simulink model "radiator model"  (R2023b)
settings: Solver=VariableStepAuto  StartTime=0.0  StopTime=1300  RelTol=1e-3  AbsTol=1e-3  EnableMultiTasking=on
PreLoadFcn:
  | %  Radiator tubes
  | n_tubes      = 20;                % Number of tubes
  | w_radiator  = 0.025;           % Radiator width [m]
  | h_tube        = 0.0015;         % Tube height [m]
  | L_tube        = 0.45;             % Tube length [m]
  | 
  | % Radiator fins
  | delta_fin     = 1e-4;           % Fin thickness [m]
  | w_fin           = 0.002;          % Fin width [m]
  | h_fin           = 0.012;            % Fin height
  | 
  | 
  | % Fluid jacket
  | Re_TLU   = [6, 8, 12, 14, 16]' .* 1e4;  % Reynolds number vector
  | Pr_TLU   = [2, 4, 6, 8, 10];                  % Prandtl number vector
  | 
  | % Air
  | rho_air          = 1.2;       % Density [kg/m^3]
  | cp_air            = 1004;   % Specific heat [J/kg/K]
  | vel_air_nom = 1;         % Nominal velocity [m/s]
  | HC_nom       = 100;     % Nominal heat transfer coefficient [W/(K*m^2)]
  | HC_min        = 10;       % Minimum heat transfer coefficient [W/(K*m^2)]
InitFcn:
  | % Radiator fins
  | n_fin_rows  = n_tubes - 1;   % Number of fin rows
  | n_fins         = n_fin_rows  * (L_tube / w_fin);   % Total number of fins
  | 
  | % Heat transfer surface area
  | area_primary = 2 * L_tube * w_radiator * (n_fin_rows) - 2 * delta_fin * w_radiator * n_fins + 2 * h_fin * w_radiator * n_fin_rows + 2 * h_tube * n_tubes * L_tube;
  | area_fins        = n_fins * (h_fin-delta_fin) * w_radiator * 2;
  | 
  | % Air
  | area_air = n_fins * h_fin * w_fin;      % Cross-sectional area [m^2]
  | 
  | % Fluid jacket
  | Nu_TLU  = 0.3.* Re_TLU .^ 0.8 * Pr_TLU .* 0.33;  %  Nusselt number table
libraries: fl_lib x13, nesl_utility x9, SimscapeFluids_lib x4
(part 1 of 3)
CloseFcn:
  | try,close(h1_EngineCoolingSystem),end
  | clear h1_EngineCoolingSystem
  | 
  | try,close(h2_EngineCoolingSystem),end
  | clear h2_EngineCoolingSystem
  | 
  | try,close(h3_EngineCoolingSystem),end
  | clear h3_EngineCoolingSystem
  | 
  | try,close(h4_EngineCoolingSystem),end
  | clear h4_EngineCoolingSystem
  | 
  | clear Eng_speed Eng_torque Fan_volt Veh_speed
  | clear n_tubes w_radiator h_tube L_tube
  | clear n_fin_rows delta_fin w_fin h_fin n_fins
  | clear area_primary area_fins
  | clear Re_TLU Pr_TLU Nu_TLU
  | clear rho_air cp_air area_air
  | clear vel_air_nom HC_nom HC_min
  | clear simlog_EngineCoolingSystem yout tout
  | clear logsout_EngineCoolingSystem
Description:
  | Engine Cooling System
settings Model: Creator=The MathWorks, Inc.  LastModifiedBy=Pranjal
settings SolverCC: AutoScaleAbsTol=off  MaxConsecutiveMinStep=2  AlgebraicLoopSolver=TrustRegion  MaxZcPerStep=1
settings DataIOCC: LimitDataPoints=on  MaxDataPoints=35000  ReturnWorkspaceOutputs=off  SignalLoggingName=logsout_EngineCoolingSystem
settings OptimizationCC: ReuseModelBlockBuffer=off  LifeSpan=inf
settings DebuggingCC: UnconnectedInputMsg=warning  UnconnectedOutputMsg=warning  UnconnectedLineMsg=warning  AllowSymbolicDim=off  PregeneratedLibrarySubsystemCodeDiagnostic=none  SFUnexpectedBacktrackingDiag=warning  SFNoUnconditionalDefaultTransitionDiag=warning  SFExecutionAtInitializationDiag=none  ArithmeticOperatorsInVariantConditions=warning
settings ModelReferenceCC: EnableRefExpFcnMdlSchedulingChecks=on  PropagateSignalLabelsOutOfModel=off
settings SFSimCC: SimUseLocalCustomCode=off  CustomCodeUndefinedFunction=UseInterfaceOnly
settings RTWCC: RTWUseLocalCustomCode=off  DLArmComputeVersion=19.05
settings CodeAppCC: StateflowObjectComments=on
settings GRTTargetCC: TargetLangStandard=C89/C90 (ANSI)
settings ConfigComp: CovMetricSettings=dw  CovSaveCumulativeToWorkspaceVar=on  CovSaveSingleToWorkspaceVar=on  CovExternalEMLEnable=off
settings SimscapeCC: SimscapeNormalizeSystem=off  SimscapeLogType=all  SimscapeLogSimulationStatistics=on  SimscapeLogName=simlog_EngineCoolingSystem  SimscapeLogDataHistory=35000

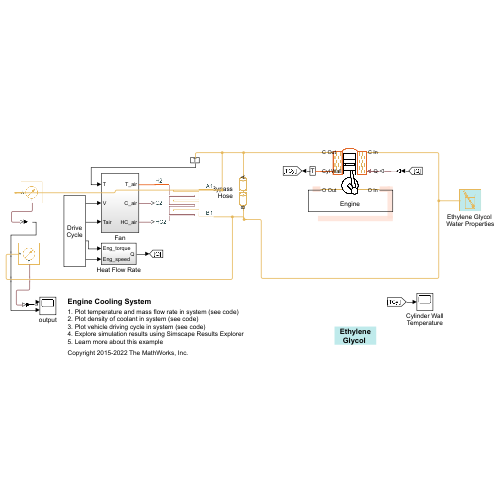
[thumbnail: Simulink's stored preview of the top-level diagram]
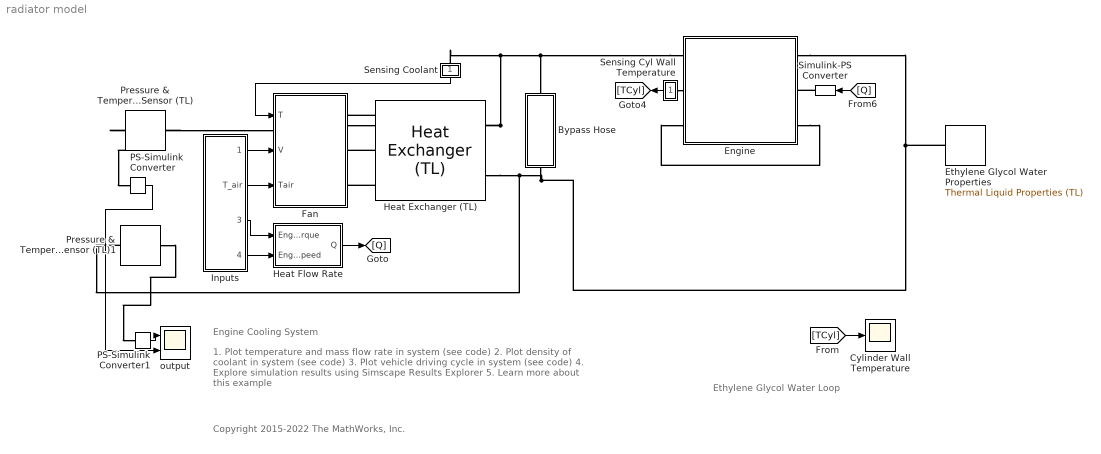
== system radiator model ==
  note: Engine Cooling System
  note: 1. Plot temperature and mass flow rate in system (see code)
      | 2. Plot density of coolant in system (see code)
      | 3. Plot vehicle driving cycle in system (see code)
      | 4. Explore simulation results using Simscape Results Explorer
      | 5. Learn more about this example
  note: Ethylene Glycol
      | Water Loop
  note: Copyright 2015-2022 The MathWorks, Inc.
  Bypass Hose : Subsystem
      mask Display: image('EngineCoolingSystemPipeImage.png');
  Cylinder Wall Temperature : Scope
  Engine : Subsystem
      mask Display: image('EngineCoolingSystemEngineImage.png');
  Ethylene Glycol Water Properties : SimscapeFluids_lib/Thermal Liquid/Utilities/Thermal Liquid Properties (TL)  fluid_list=3  concentration_param_EG=1  concentration_param_PG=1  c_mass_SW=3.5e-3  c_mass_EG=0.1  c_mass_PG=0.1  c_mass_GL=0.1  c_vol_EG=0.5  c_vol_PG=0.1  beta_const_EG=2.1791 GPa  beta_const_PG=2.1791 GPa  beta_const_GL=2.1791 GPa  p_min_EG=0.01 MPa  p_min_PG=0.01 MPa  p_min_GL=0.01 MPa  p_max_EG=50 MPa  p_max_PG=50 MPa  p_max_GL=50 MPa  p_atm=0.101325 MPa  properties_range_check=simscape.enum.assert.action.error
  Fan : Subsystem
  Heat Exchanger (TL) : SimscapeFluids_lib/Fluid Network Interfaces/Heat Exchangers/Heat Exchanger (TL)  hex_type=fluids.interfaces.enum.flow_arrangement_spec.cross_flow  shell_num=1  cross_type=fluids.interfaces.enum.cross_flow_heat_exchanger_TL_spec.mixed_mixed  NTU_TLU=[.5, 1, 2, 3, 4, 5]  CR_TLU=[0, .25, .5, .75, 1]  eff_TLU=[.3, .3, .3, .3, .3; .6, .55, .5, .47, .43; .85, .76, .68, .61, .55; .94, .83, .72, .65, .58; .98, .86, .75, .66, .58; .99, .86, .75, .66, .58]  R_wall=1.6e-4 K/W  min_flow_area_1=19084.8 cm^2  Dh_press_1=25.57598 cm  liquid_volume_1=22901.76 cm^3  Re_lam_1=2000  Re_tur_1=4000  pressure_loss_spec_1=fluids.interfaces.enum.pressure_loss_spec.constant  pressure_loss_coeff_1=0.1  length_press_1=1 m  length_add_1=0.1 m  roughness_1=15e-6 m  Re_friction_TLU_1=[400, 1000, 1500, 3000, 4000, 6000, 10000, 20000, 40000, 60000, 100000, 100000000]  friction_factor_TLU_1=[.264, .112, .071, .0417, .0387, .0268, .025, .0232, .0226, .022, .0214, .0214]  shape_factor_1=64  Re_Euler_TLU_1=[50, 500, 1000, 2000]  Euler_TLU_1=[4.4505, .6864, .4791, .3755]  heat_transfer_spec_1=fluids.interfaces.enum.heat_transfer_spec.constant  heat_transfer_area_1=3581.76 cm^2  heat_coeff_1=4000 W/(K*m^2)  length_heat_1=1 m  Nu_lam_1=3.66  Re_Colburn_TLU_1=[100, 150, 1000]  Colburn_factor_TLU_1=[.019, .013, .002]  Re_Nu_TLU_1=[100, 150, 1000]  Pr_Nu_TLU_1=[1, 10]  Nu_TLU_1=[3.72, 4.21; 3.75, 4.44; 4.21, 7.15]  fouling_factor_1=0 K*m^2/W  min_heat_coeff_1=10 W/(K*m^2)  heat_transfer_area_2=0.17 m^2  fouling_factor_2=1e-4 K*m^2/W  min_heat_coeff_2=0.02 W/(K*m^2)  dynamic_compressibility_1=simscape.enum.onoff.on  T0_1=293.15 K  p0_1=1 atm  mdot1_TLU=[.3, .5, .6, .7, 1, 1.4, 1.9, 2.3] kg/s  mdot2_TLU=[.3, .5, 1, 1.3, 1.7, 2, 2.6, 3.3] kg/s  SD_TLU=[.324, .3533, .404, .4253, .4333, .4373, .4453, .4533; .3813, .424, .496, .5307, .544, .5547, .5693, .5787; .4267, .4827, .5813, .6173, .6413, .6573, .672, .6827; .4613, .528, .64, .6987, .7267, .7467, .7707, .7853; .5533, .6467, .8227, .928, .9853, 1.0187, 1.0653, 1.0973; .58, .688, .8853, 1.0147, 1.08, 1.124, 1.176, 1.2147; .624, .7467, .992, 1.148, 1.244, 1.304, 1.3773, 1.4267; .656, .7907, 1.0667, 1.26, 1.376, 1.452, 1.548, 1.612] kW/K  Q_check=fluids.interfaces.enum.SD_max_check.warning  mdot_dp_TLU_1=[.3, .5, 1, 1.5, 2, 2.5] kg/s  p_diff_TLU_1=[3, 5, 10, 25, 35, 50] * 1e-3 MPa  T_ref_in_1=293.15 K  p_ref_in_1=0.101325 MPa  mdot_threshold_1=1e-3 kg/s  area_1=0.01 m^2
      settings: InternalSimscapePortConfiguration="{\"Bottom\":[],\"Left\":[{\"id\":\"A1\",\"label\":\"A1\",\"type\":\"foundation.thermal_liquid.thermal_liquid\"},{\"id\":\"B1\",\"label\":\"B1\",\"type\":\"foundation.thermal_liquid.thermal_liquid\"}],\"Right\":[{\"id\":\"H2\",\"label\":\"H2\",\"type\":\"foundation.thermal.thermal\"},{\"id\":\"C2\",\"label\":\"C2\",\"type\":\"input\"},{\"id\":\"HC2\",\"label\":\"HC2\",\"type\":\"input\"}],\"Top\":[]}"
  Heat Flow Rate : Subsystem
  Inputs : Subsystem
      mask Display: disp('Drive\nCycle')
  PS-Simulink Converter : nesl_utility/PS-Simulink Converter  PhysicalDomain=network_engine_domain  SubClassName=ps_output  LeftPortType=input  RightPortType=output  PseudoPeriodic=off  Frequencies=[]  VectorFormat=inherit  Unit=inherit  AffineConversion=off
  PS-Simulink Converter1 : nesl_utility/PS-Simulink Converter  PhysicalDomain=network_engine_domain  SubClassName=ps_output  LeftPortType=input  RightPortType=output  PseudoPeriodic=off  Frequencies=[]  VectorFormat=inherit  Unit=inherit  AffineConversion=off
  Pressure & Temperature Sensor (TL) : fl_lib/Thermal Liquid/Sensors/Pressure & Temperature Sensor (TL)  reference=foundation.enum.MeasurementReference.absolute  pressure=false  pressure_spec=foundation.enum.PressureMeasementSpec.Absolute  temperature=true
      settings: InternalSimscapePortConfiguration="{\"Bottom\":[{\"id\":\"T\",\"label\":\"T\",\"type\":\"output\"}],\"Left\":[{\"id\":\"A\",\"label\":\"A\",\"type\":\"foundation.thermal_liquid.thermal_liquid\"}],\"Right\":[],\"Top\":[]}"
  Pressure & Temperature Sensor (TL)1 : fl_lib/Thermal Liquid/Sensors/Pressure & Temperature Sensor (TL)  reference=foundation.enum.MeasurementReference.absolute  pressure=false  pressure_spec=foundation.enum.PressureMeasementSpec.Absolute  temperature=true
      settings: InternalSimscapePortConfiguration="{\"Bottom\":[{\"id\":\"T\",\"label\":\"T\",\"type\":\"output\"}],\"Left\":[{\"id\":\"A\",\"label\":\"A\",\"type\":\"foundation.thermal_liquid.thermal_liquid\"}],\"Right\":[],\"Top\":[]}"
  Sensing Cyl Wall Temperature : Subsystem
      mask Display: disp('T');
  Sensing Coolant : Subsystem
      mask Display: disp('T');
  Simulink-PS Converter : nesl_utility/Simulink-PS Converter  PhysicalDomain=network_engine_domain  SubClassName=ps_input  LeftPortType=input  RightPortType=output  PseudoPeriodic=off  Frequencies=[]  NoiseDistribution=none  NoiseParameters=[]  Unit=W  AffineConversion=off  FilteringAndDerivatives=provide  SimscapeFilterOrder=1  InputFilterTimeConstant=0.001  UdotUserProvided=0
  output : Scope  NumInputPorts=2
  wires:
  Inputs/4(Eng_speed) -> Heat Flow Rate/2(Eng_speed)
  Inputs/3(Eng_torque) -> Heat Flow Rate/1(Eng_torque)
  Inputs/2(T_air) -> Fan/3(Tair)
  Sensing Coolant/1(Out1) -> Fan/1(T)
  Sensing Cyl Wall Temperature/1(Out1) -> [TCyl]
  [TCyl] -> Cylinder Wall Temperature/1
  [Q] -> Simulink-PS Converter/1
  Inputs/1(Veh_speed) -> Fan/2(V)
  Heat Flow Rate/1(Q) -> [Q]
  PS-Simulink Converter/1 -> output/2
  PS-Simulink Converter1/1 -> output/1
  connections:
  Engine/RConn1 -- Sensing Coolant/LConn1 -- Pressure & Temperature Sensor (TL)/LConn1 -- Heat Exchanger (TL)/LConn1 -- Bypass Hose/LConn1
  Sensing Cyl Wall Temperature/LConn1 -- Engine/RConn2
  Engine/LConn1 -- Pressure & Temperature Sensor (TL)1/LConn1 -- Heat Exchanger (TL)/LConn2 -- Bypass Hose/RConn1 -- Ethylene Glycol Water Properties/RConn1
  Simulink-PS Converter/RConn1 -- Engine/LConn2
  Engine/LConn3 -- Engine/RConn3
  Heat Exchanger (TL)/RConn2 -- Fan/RConn2
  Heat Exchanger (TL)/RConn1 -- Fan/RConn1
  Heat Exchanger (TL)/RConn3 -- Fan/RConn3
  Pressure & Temperature Sensor (TL)/RConn1 -- PS-Simulink Converter/LConn1
  Pressure & Temperature Sensor (TL)1/RConn1 -- PS-Simulink Converter1/LConn1

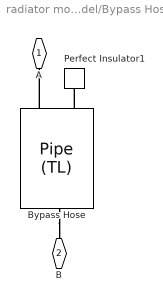
== system radiator model/Bypass Hose ==
  Bypass Hose : SimscapeFluids_lib/Thermal Liquid/Pipes & Fittings/Pipe (TL)  dynamic_compressibility=simscape.enum.onoff.on  inertia=simscape.enum.onoff.off  num_segments=1  pipe_length=1 m  cross_section_geometry=fluids.thermal_liquid.pipes_fittings.enum.CrossSectionGeometry.Custom  pipe_diameter=0.1 m  pipe_inner_diameter=0.05 m  pipe_outer_diameter=0.1 m  pipe_width=0.1 m  pipe_height=0.1 m  pipe_major_axis=0.1 m  pipe_minor_axis=0.05 m  pipe_side=0.1 m  pipe_angle=30 deg  area=pi*0.01^2 m^2  Dh=0.02 m  elevation_spec=foundation.enum.constant_variable.constant  elevation_gain=0 m  gravity_spec=foundation.enum.constant_variable.constant  g=9.81 m/s^2  pressure_loss_spec=fluids.thermal_liquid.pipes_fittings.enum.PressureLossSpec.Haaland  local_pressure_loss_spec=fluids.thermal_liquid.pipes_fittings.enum.LocalLossSpec.AggregateLength  length_add=5 m  loss_coefficient=0.1  roughness_spec=fluids.thermal_liquid.pipes_fittings.enum.RoughnessSpec.Custom  roughness=1.5e-5 m  Re_friction_TLU=[ 400 1000 1.5e+3 3e+3 4e+3 6e+3 1e+4 2e+4 4e+4 6e+4 1e+5 1e+8 ]  friction_factor_TLU=[ 0.264 0.112 0.07099999999999999 0.0417 0.0387 0.0268 0.025 0.0232 0.0226 0.022 0.0214 0.0214 ]  Re_lam=2e+3  Re_tur=4e+3  shape_factor=64  mdot_nominal=[ 0.1 1 ] kg/s  p_diff_nominal=[ 0.001 0.01 ] MPa  mdot_threshold=1e-6 kg/s  wall_spec=fluids.thermal_liquid.pipes_fittings.enum.wall_spec.rigid  vol_expansion_spec=fluids.thermal_liquid.pipes_fittings.enum.VolumeExpansionSpec.Diameter  area_pressure_gain=1e-6 m^2/MPa  static_pressure_TLU=[.1, 1] MPa  area_pressure_gain_TLU=[1e-05, 1.1e-05] m^2  material_behavior_spec=fluids.thermal_liquid.pipes_fittings.enum.PipeMaterialBehavior.Linear  diameter_pressure_gain=1e-6 m/MPa  wall_thickness=0.05 m  elastic_modulus=69 GPa  stress_TLU=[276, 310] MPa  strain_TLU=[.004, .02]  stress_assert_action=simscape.enum.assert.action.none  stress_max=400 MPa  poisson_ratio=0.33  wall_time_constant=0.01 s  thermal_expansion=false  alpha_L_wall=24 um/(deltaK*m)  thermal_expansion_Tref=293.15 K  heat_transfer_spec=fluids.thermal_liquid.pipes_fittings.enum.HeatTransferSpec.Gnielinski  mdot_nominal_heat=[ 0.1 1 ] kg/s  T_in_nominal=[ 293.15 293.15 ] K  T_out_nominal=[ 300 300 ] K  p_in_nominal_heat=[ 0.101325 0.101325 ] MPa  T_wall_nominal=[ 303.15 303.15 ] K  a_coeff=0.023  b_Re_power=0.8  c_Pr_power=0.4  Nu_lam=3.66  Re_Colburn_TLU=[ 100 150 1000 ]  Colburn_factor_TLU=[ 0.019 0.013 0.002 ]  Re_Nu_TLU=[ 100 150 1000 ]  Pr_Nu_TLU=[ 1 10 ]  Nu_TLU=[ 3.72 4.21; 3.75 4.44; 4.21 7.15 ]  p0_vec=0.101325 MPa  T0_vec=303.15 K  mdot0=0.1 kg/s
  Perfect Insulator1 : fl_lib/Thermal/Thermal Elements/Perfect Insulator  T_specify=off  T_priority=None  T=0 K  T_nominal_specify=off  T_nominal_unit=K  T_nominal_value=1
  A : PMIOPort  Side=Left
  B : PMIOPort  Port=2  Side=Right
  connections:
  Bypass Hose/LConn2 -- Perfect Insulator1/LConn1
  Bypass Hose/RConn1 -- B/RConn1
  Bypass Hose/LConn1 -- A/RConn1

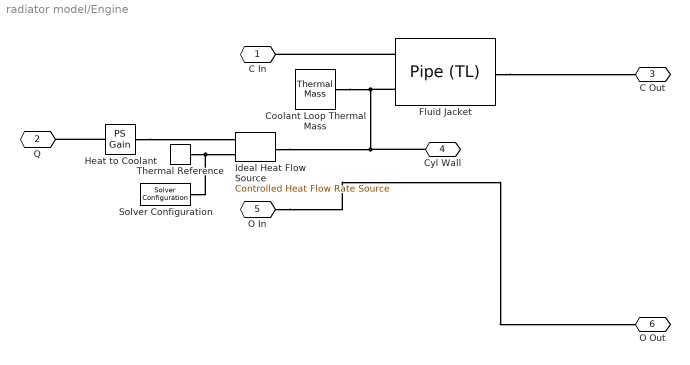
== system radiator model/Engine ==
  Coolant Loop Thermal Mass : fl_lib/Thermal/Thermal Elements/Thermal Mass  mass_type=foundation.enum.constant_variable.constant  mass=0.2 kg  sp_heat=800 J/(K*kg)  mass_min=1e-6 kg  num_ports=foundation.enum.numPorts2.one  m_specify=off  m_priority=High  m=1 kg  m_nominal_specify=off  m_nominal_unit=kg  m_nominal_value=1  T_specify=on  T_priority=High  T=30 degC  T_nominal_specify=off  T_nominal_unit=K  T_nominal_value=1  Q_specify=off  Q_priority=High  Q=0 J/s  Q_nominal_specify=off  Q_nominal_unit=J/s  Q_nominal_value=1
  Fluid Jacket : SimscapeFluids_lib/Thermal Liquid/Pipes & Fittings/Pipe (TL)  dynamic_compressibility=simscape.enum.onoff.on  inertia=simscape.enum.onoff.off  num_segments=1  pipe_length=500 cm  cross_section_geometry=fluids.thermal_liquid.pipes_fittings.enum.CrossSectionGeometry.Custom  pipe_diameter=0.1 m  pipe_inner_diameter=0.05 m  pipe_outer_diameter=0.1 m  pipe_width=0.1 m  pipe_height=0.1 m  pipe_major_axis=0.1 m  pipe_minor_axis=0.05 m  pipe_side=0.1 m  pipe_angle=30 deg  area=500 mm^2  Dh=10 mm  elevation_spec=foundation.enum.constant_variable.constant  elevation_gain=0 m  gravity_spec=foundation.enum.constant_variable.constant  g=9.81 m/s^2  pressure_loss_spec=fluids.thermal_liquid.pipes_fittings.enum.PressureLossSpec.Haaland  local_pressure_loss_spec=fluids.thermal_liquid.pipes_fittings.enum.LocalLossSpec.AggregateLength  length_add=1 m  loss_coefficient=0.1  roughness_spec=fluids.thermal_liquid.pipes_fittings.enum.RoughnessSpec.Custom  roughness=1.5e-5 m  Re_friction_TLU=[ 400 1000 1.5e+3 3e+3 4e+3 6e+3 1e+4 2e+4 4e+4 6e+4 1e+5 1e+8 ]  friction_factor_TLU=[ 0.264 0.112 0.07099999999999999 0.0417 0.0387 0.0268 0.025 0.0232 0.0226 0.022 0.0214 0.0214 ]  Re_lam=2e+3  Re_tur=4e+3  shape_factor=64  mdot_nominal=[ 0.1 1 ] kg/s  p_diff_nominal=[ 0.001 0.01 ] MPa  mdot_threshold=1e-6 kg/s  wall_spec=fluids.thermal_liquid.pipes_fittings.enum.wall_spec.rigid  vol_expansion_spec=fluids.thermal_liquid.pipes_fittings.enum.VolumeExpansionSpec.Diameter  area_pressure_gain=1e-6 m^2/MPa  static_pressure_TLU=[.1, 1] MPa  area_pressure_gain_TLU=[1e-05, 1.1e-05] m^2  material_behavior_spec=fluids.thermal_liquid.pipes_fittings.enum.PipeMaterialBehavior.Linear  diameter_pressure_gain=1e-6 m/MPa  wall_thickness=0.05 m  elastic_modulus=69 GPa  stress_TLU=[276, 310] MPa  strain_TLU=[.004, .02]  stress_assert_action=simscape.enum.assert.action.none  stress_max=400 MPa  poisson_ratio=0.33  wall_time_constant=0.01 s  thermal_expansion=false  alpha_L_wall=24 um/(deltaK*m)  thermal_expansion_Tref=293.15 K  heat_transfer_spec=fluids.thermal_liquid.pipes_fittings.enum.HeatTransferSpec.TabulatedNusselt  mdot_nominal_heat=[ 0.1 1 ] kg/s  T_in_nominal=[ 293.15 293.15 ] K  T_out_nominal=[ 300 300 ] K  p_in_nominal_heat=[ 0.101325 0.101325 ] MPa  T_wall_nominal=[ 303.15 303.15 ] K  a_coeff=0.023  b_Re_power=0.8  c_Pr_power=0.4  Nu_lam=3.66  Re_Colburn_TLU=[ 100 150 1000 ]  Colburn_factor_TLU=[ 0.019 0.013 0.002 ]  Re_Nu_TLU=Re_TLU  Pr_Nu_TLU=Pr_TLU  Nu_TLU=Nu_TLU  p0_vec=0.101325 MPa  T0_vec=303.15 K  mdot0=0.1 kg/s
  Heat to Coolant : fl_lib/Physical Signals/Functions/PS Gain  gain=0.5
      settings: AttributesFormatString=%<gain>
  Ideal Heat Flow Source : fl_lib/Thermal/Thermal Sources/Controlled Heat Flow Rate Source
  Solver Configuration : nesl_utility/Solver Configuration  PhysicalDomain=network_engine_domain  SubClassName=solver  LeftPortType=input  RightPortType=generic  Tones=[]  Harmonics=[]  SimulateNoise=off  Profile=off  UseLocalSampling=off  EnableSwitchedLinearOptims=on  FrequencyDomain=off  UseCCode=off  RelTol=0.001  AbsTol=1e-06  MinStep=1e-09  ToWorkspace=off  RevertToSquareIcSolve=off  NumHomotopyIterations=100  PhasorMode=off  PhasorModeNumHarmonics=1  ConsistencySolver=NEWTON_XTOL_AFTER_FTOL  IndexReductionMethod=DerivativeReplacement  DoDC=off  ResidualTolerance=1e-9  ConsistencyTolSource=GLOBAL  ConsistencyAbsTol=0.001  ConsistencyRelTol=0.001  ConsistencyTolFactor=0.001  UseLocalSolver=off  LocalSolverChoice=NE_BACKWARD_EULER_ADVANCER  ResolveIndetEquations=on  FunctionEvalNumThread=1  LocalSolverSampleTime=1  DoFixedCost=off  MaxNonlinIter=3  MaxModeIter=2  ComputeImpulses=off  ImpulseIterations=2  LinearAlgebra=auto  LinearAlgebraNumThread=0  EquationFormulation=NE_TIME_EF  DelaysMemoryBudget=1024  AutomaticFiltering=on  FilteringTimeConstant=0.001  PartitionStorageMethod=AS_NEEDED  PartitionMemoryBudget=1024  PartitionMethod=FAST  MultibodyUseLocalSolver=off  MultibodyLocalSolverChoice=ODE1  MultibodyLocalSolverSampleTime=0.001
  Thermal Reference : fl_lib/Thermal/Thermal Elements/Thermal Reference
  C In : PMIOPort  Side=Left
  Q : PMIOPort  Port=2  Side=Left
  C Out : PMIOPort  Port=3  Side=Right
  Cyl Wall : PMIOPort  Port=4  Side=Right
  O In : PMIOPort  Port=5  Side=Left
  O Out : PMIOPort  Port=6  Side=Right
  connections:
  Fluid Jacket/RConn1 -- C Out/RConn1
  Coolant Loop Thermal Mass/LConn1 -- Fluid Jacket/LConn2 -- Ideal Heat Flow Source/LConn1 -- Cyl Wall/RConn1
  Thermal Reference/LConn1 -- Solver Configuration/RConn1 -- Ideal Heat Flow Source/RConn2
  Fluid Jacket/LConn1 -- C In/RConn1
  O In/RConn1 -- O Out/RConn1
  Heat to Coolant/LConn1 -- Q/RConn1
  Heat to Coolant/RConn1 -- Ideal Heat Flow Source/RConn1

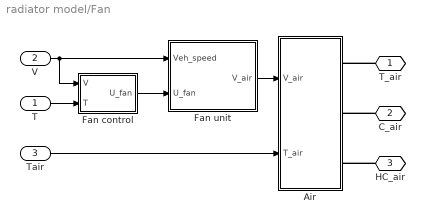
== system radiator model/Fan ==
  T : Inport
  V : Inport  Port=2
  Tair : Inport  Port=3
  Air : Subsystem
  Fan control : Subsystem  mask(2-Level Fan Controller){T_level1=[97 94], T_level2=[105 102]}
      mask prompts: T_level1 "Level 1 temperature"; T_level2 "Level 2 temperature"
      mask help: The primary and secondary fan control temperature ranges are defined by Level 1 temperature vector and Level 2 temperature vector, respectively.
  Fan unit : Subsystem
  T_air : PMIOPort  Side=Right
  C_air : PMIOPort  Port=2  Side=Right
  HC_air : PMIOPort  Port=3  Side=Right
  wires:
  Tair/1 -> Air/2(T_air)
  V/1 -> Fan control/1(V), Fan unit/1(Veh_speed)
  Fan unit/1(V_air) -> Air/1(V_air)
  Fan control/1(U_fan) -> Fan unit/2(U_fan)
  T/1 -> Fan control/2(T)
  connections:
  T_air/RConn1 -- Air/RConn1
  C_air/RConn1 -- Air/RConn2
  HC_air/RConn1 -- Air/RConn3

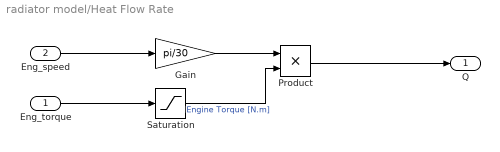
== system radiator model/Heat Flow Rate ==
  Eng_torque : Inport
  Eng_speed : Inport  Port=2
  Gain : Gain  Gain=pi/30
  Product : Product
  Saturation : Saturate  UpperLimit=inf  LowerLimit=0
  Q : Outport  VectorParamsAs1DForOutWhenUnconnected=off
  wires:
  Saturation/1 -> Product/2  "Engine Torque [N.m]"
  Eng_torque/1 -> Saturation/1
  Product/1 -> Q/1
  Gain/1 -> Product/1
  Eng_speed/1 -> Gain/1
